simulink model "TargetPosVel"  (R2024b)
settings: Solver=ode4  StartTime=0.0  StopTime=stopTime  FixedStep=timeStep  RelTol=1e-3
values from neighbouring files (symbols this model uses):
  c = 299792458    [FMC.m]
  CD = 2.2    [FMC.m]
  dayValue = 1    [FMC.m]    (also in validation.m)
  dimx = 226.3/1000    (= 0.2263)    [FMC.m]
  dimz = 360/1000    (= 0.36)    [FMC.m]
  FL = 50e-3    (= 0.05)    [FMC.m]
  fps = 1/timeStep    (= 20)    [FMC.m]
  hourValue = 12    [FMC.m]    (also in validation.m)
  I = [Ixx Ixy Ixz; Ixy Iyy Iyz; Ixz Iyz Izz]    [FMC.m]
  I_W = [I_w 0 0; 0 I_w 0; 0 0 I_w]    [FMC.m]
  kd = 0.022    [FMC.m]
  kq = 0.0032    [FMC.m]
  L_pixel = 4.8e-6    (= 4.8e-06)    [FMC.m]
  max_h = I_w*max_speed    (= 0.00954258768528)    [FMC.m]
  max_t = 2e-3    (= 0.002)    [FMC.m]
  minuteValue = 0    [FMC.m]    (also in validation.m)
  mu_E = 3.986004418e14    (= 398600441800000)    [FMC.m]
  Omega_E = 7.2921159e-5    (= 7.2921159e-05)    [FMC.m]
  P0_Kfilter = blkdiag(eye(3), eye(3))    [FMC.m]
  Phi = 1358    [FMC.m]
  pointing_body = [0,0,1]    [FMC.m]
  q = 0.6    [FMC.m]
  Q_b = 0.05*eye(3)    [FMC.m]
  Q_LoS = 0.1*eye(3)    [FMC.m]
  quat0 = [0.6387; -0.3737; 0.6003; 0.3034]    [FMC.m]
  R_E = 6378*1000    (= 6378000)    [FMC.m]
  R_meas = norm(LoS_0)*L_pixel*fps/FL*Q_b    [FMC.m]
  rand_vec = rand_vec/norm(rand_vec)    [FMC.m]
  rcp = [0.013 0.02 0.05]    [FMC.m]
  res_dipole = 0.05    [FMC.m]
  secondValue = 0    [FMC.m]    (also in validation.m)
  sma = R_E + H    (= 6628000)    [FMC.m]
  timeStep = 0.05    [FMC.m]
  w0 = [w0x; w0y; w0z]    [FMC.m]
  x0_Kfilter = [LoS_0,;b_0]    [FMC.m]
  yearValue = 2025    [FMC.m]    (also in validation.m)
undefined symbols (not defined in the file or in its folder): IAU, WMM2020
libraries: aerolibtransform2 x14, aerolibutil x13, matrix_library x12, vrlib x5, sharedtransform x2, sharedTrackingLibrary x1, aerolibatmos2 x1, aerolibgravity2 x1, sensorgpslib x1, visionsources x1
(part 1 of 2)
settings Model: Creator=nicolasgagliardi  LastModifiedBy=nicolasgagliardi

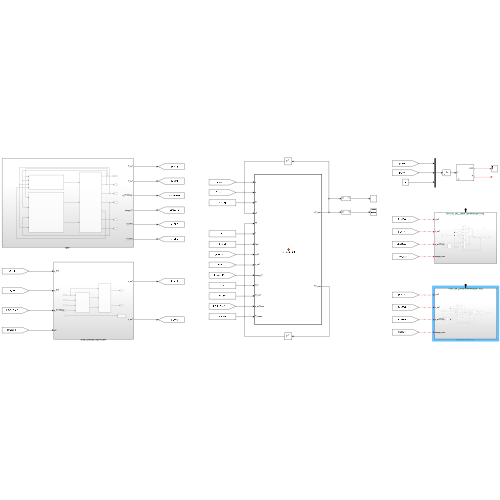
[thumbnail: Simulink's stored preview of the top-level diagram]
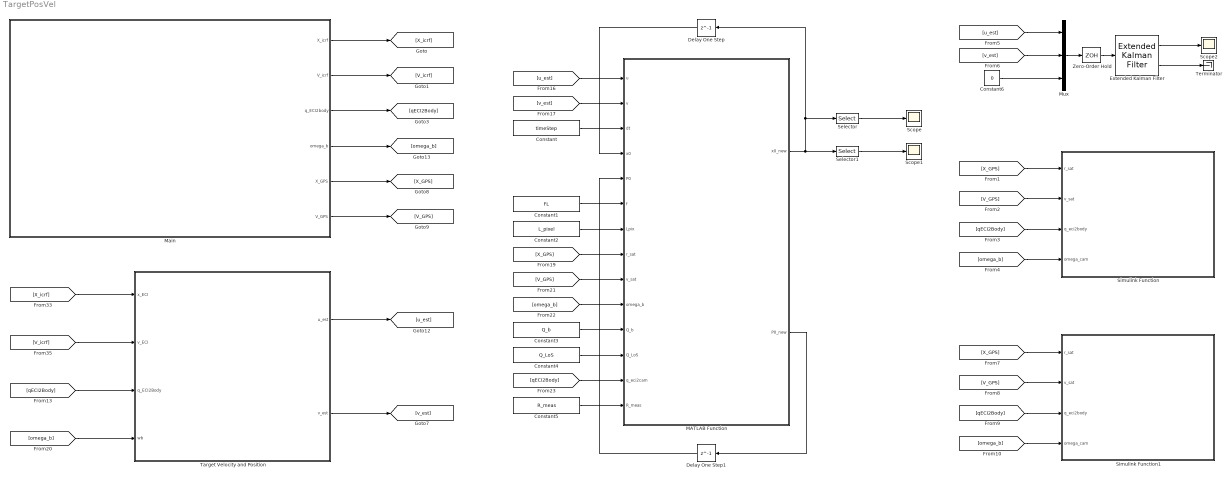
== system TargetPosVel ==
  Constant : Constant  Value=timeStep
  Constant1 : Constant  Value=FL
  Constant2 : Constant  Value=L_pixel
  Constant3 : Constant  Value=Q_b
  Constant4 : Constant  Value=Q_LoS
  Constant5 : Constant  Value=R_meas
  Constant6 : Constant  Value=0
  Delay One Step : Delay  DelayLength=1  InitialCondition=x0_Kfilter  SampleTime=timeStep
  Delay One Step1 : Delay  DelayLength=1  InitialCondition=P0_Kfilter  SampleTime=timeStep
  Extended Kalman Filter : sharedTrackingLibrary/Extended Kalman Filter  StateTransitionFcn=state_dynamics  HasStateTransitionJacobianFcn=off  HasAdditiveProcessNoise=Additive  ProcessNoise=Q_LoS  HasTimeVaryingProcessNoise=off  HasStateTransitionFcnExtraArgument=0  InitialState=x0_Kfilter(1:3)  InitialStateCovariance=P0_Kfilter(1:3,1:3)  MeasurementFcn1=measurements  HasMeasurementJacobianFcn1=off  HasMeasurementEnablePort1=off  HasAdditiveMeasurementNoise1=Additive  MeasurementNoise1=R_meas  HasTimeVaryingMeasurementNoise1=off  HasMeasurementFcnExtraArgument1=0  HasMeasurementWrapping1=off  MeasurementFcn2=myMeasurementFcn  HasMeasurementJacobianFcn2=off  HasMeasurementEnablePort2=off  HasAdditiveMeasurementNoise2=Additive  MeasurementNoise2=1  HasTimeVaryingMeasurementNoise2=off  HasMeasurementFcnExtraArgument2=0  HasMeasurementWrapping2=off  MeasurementFcn3=myMeasurementFcn  HasMeasurementJacobianFcn3=off  HasMeasurementEnablePort3=off  HasAdditiveMeasurementNoise3=Additive  MeasurementNoise3=1  HasTimeVaryingMeasurementNoise3=off  HasMeasurementFcnExtraArgument3=0  HasMeasurementWrapping3=off  MeasurementFcn4=myMeasurementFcn  HasMeasurementJacobianFcn4=off  HasMeasurementEnablePort4=off  HasAdditiveMeasurementNoise4=Additive  MeasurementNoise4=1  HasTimeVaryingMeasurementNoise4=off  HasMeasurementFcnExtraArgument4=0  HasMeasurementWrapping4=off  MeasurementFcn5=myMeasurementFcn  HasMeasurementJacobianFcn5=off  HasMeasurementEnablePort5=off  HasAdditiveMeasurementNoise5=Additive  MeasurementNoise5=1  HasTimeVaryingMeasurementNoise5=off  HasMeasurementFcnExtraArgument5=0  HasMeasurementWrapping5=off  EnableMultirate=off  StateTransitionFcnSampleTime=1  MeasurementFcn1SampleTime=1  MeasurementFcn2SampleTime=1  MeasurementFcn3SampleTime=1  MeasurementFcn4SampleTime=1  MeasurementFcn5SampleTime=1  UseCurrentEstimator=on  OutputStateCovariance=on  DataType=double  SampleTime=timeStep  NumberOfMeasurements=1
  MATLAB Function : MATLAB Function  TreatAsAtomicUnit=on
  Main : Subsystem
  Mux : Mux  Inputs=3
  Scope : Scope
  Scope1 : Scope
  Scope2 : Scope
  Selector : Selector  InputPortWidth=6  IndexOptions=Index vector (dialog)  Indices=[1 2 3]  OutputSizes=1
  Selector1 : Selector  InputPortWidth=6  IndexOptions=Index vector (dialog)  Indices=[4 5 6]  OutputSizes=1
  Simulink Function : Subsystem  TreatAsAtomicUnit=on
  Simulink Function1 : Subsystem  TreatAsAtomicUnit=on
  Target Velocity and Position : Subsystem
  Terminator : Terminator
  Zero-Order Hold : ZeroOrderHold  SampleTime=timeStep
  wires:
  [qECI2Body] -> Target Velocity and Position/3(q_ECI2Body)
  [omega_b] -> Target Velocity and Position/4(wb)
  [V_icrf] -> Target Velocity and Position/2(v_ECI)
  [X_icrf] -> Target Velocity and Position/1(x_ECI)
  Main/1(X_icrf) -> [X_icrf]
  Main/3(q_ECI2body) -> [qECI2Body]
  Main/4(omega_b) -> [omega_b]
  Main/2(V_icrf) -> [V_icrf]
  Target Velocity and Position/2(v_est) -> [v_est]
  Target Velocity and Position/1(u_est) -> [u_est]
  [u_est] -> MATLAB Function/1(u)
  [v_est] -> MATLAB Function/2(v)
  Constant/1 -> MATLAB Function/3(dt)
  [X_GPS] -> MATLAB Function/8(r_sat)
  [V_GPS] -> MATLAB Function/9(v_sat)
  [omega_b] -> MATLAB Function/10(omega_b)
  [qECI2Body] -> MATLAB Function/13(q_eci2cam)
  Constant2/1 -> MATLAB Function/7(Lpix)
  Constant1/1 -> MATLAB Function/6(f)
  MATLAB Function/1(x0_new) -> Delay One Step/1, Selector/1, Selector1/1
  MATLAB Function/2(P0_new) -> Delay One Step1/1
  Delay One Step/1 -> MATLAB Function/4(x0)
  Delay One Step1/1 -> MATLAB Function/5(P0)
  Main/5(X_GPS) -> [X_GPS]
  Main/6(V_GPS) -> [V_GPS]
  Constant3/1 -> MATLAB Function/11(Q_b)
  Constant4/1 -> MATLAB Function/12(Q_LoS)
  Constant5/1 -> MATLAB Function/14(R_meas)
  Selector/1 -> Scope/1
  Selector1/1 -> Scope1/1
  [X_GPS] -> Simulink Function/1(r_sat)
  [V_GPS] -> Simulink Function/2(v_sat)
  [qECI2Body] -> Simulink Function/3(q_eci2body)
  [omega_b] -> Simulink Function/4(omega_cam)
  Mux/1 -> Zero-Order Hold/1
  [X_GPS] -> Simulink Function1/1(r_sat)
  [V_GPS] -> Simulink Function1/2(v_sat)
  [qECI2Body] -> Simulink Function1/3(q_eci2body)
  [omega_b] -> Simulink Function1/4(omega_cam)
  Extended Kalman Filter/2 -> Terminator/1
  Extended Kalman Filter/1 -> Scope2/1
  Constant6/1 -> Mux/3
  [v_est] -> Mux/2
  [u_est] -> Mux/1
  Zero-Order Hold/1 -> Extended Kalman Filter/1

== system TargetPosVel/Main ==
  Control Torques : Subsystem
  Environmental Torques : Subsystem
  Subsystem : Subsystem
  X_icrf : Outport
  V_icrf : Outport  Port=2
  q_ECI2body : Outport  Port=3
  omega_b : Outport  Port=4
  X_GPS : Outport  Port=5
  V_GPS : Outport  Port=6
  wires:
  Subsystem/1(X_icrf) -> Environmental Torques/1(X_icrf), Control Torques/1(r_ECI), X_icrf/1
  Subsystem/2(V_icrf) -> Environmental Torques/2(V_icrf), Control Torques/2(v_ECI), V_icrf/1
  Subsystem/3(q_ECI2body) -> q_ECI2body/1, Environmental Torques/3(qECI2body), Control Torques/4(q_ECI2body)
  Subsystem/4(omega_b) -> omega_b/1, Control Torques/3(omega_b)
  Subsystem/5(t_JD) -> Environmental Torques/4(t_JD)
  Subsystem/6(X_GPS) -> X_GPS/1
  Subsystem/7(V_GPS) -> V_GPS/1
  Control Torques/1(h) -> Subsystem/2(h_rw)
  Control Torques/2(dh_dt) -> Subsystem/3(hdot_rw)
  Environmental Torques/1(T_tot) -> Subsystem/1(T_dist)

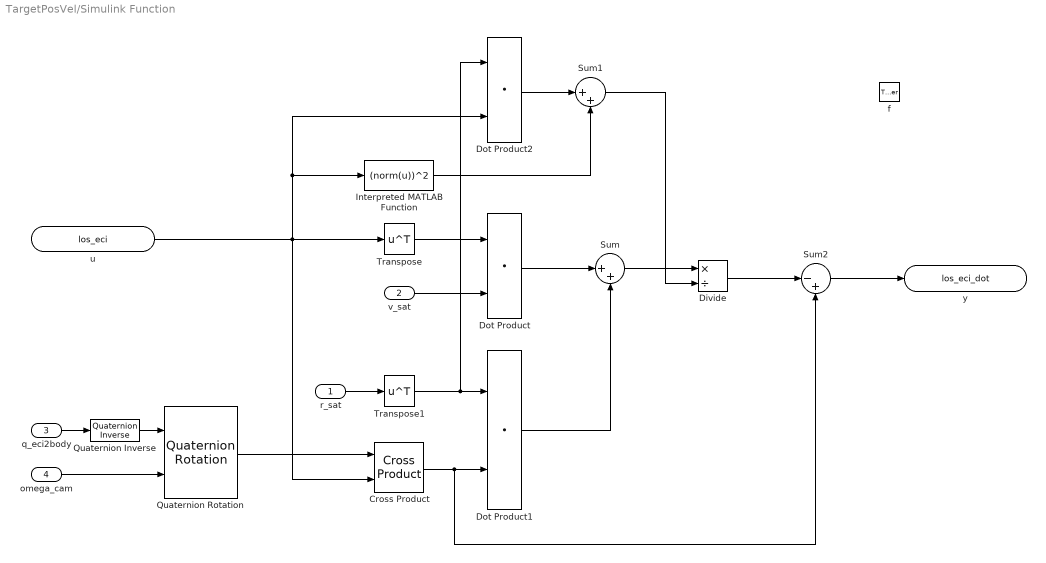
== system TargetPosVel/Simulink Function ==
  r_sat : Inport
  v_sat : Inport  Port=2
  q_eci2body : Inport  Port=3
  omega_cam : Inport  Port=4
  f : TriggerPort  TriggerType=function-call  IsSimulinkFunction=on  FunctionName=state_dynamics  FunctionVisibility=scoped  VariantControl=(inherit)
  Cross Product : matrix_library/Cross Product
  Divide : Product  Inputs=*/
  Dot Product : DotProduct  OutDataTypeStr=Inherit: Inherit via internal rule
  Dot Product1 : DotProduct  OutDataTypeStr=Inherit: Inherit via internal rule
  Dot Product2 : DotProduct  OutDataTypeStr=Inherit: Inherit via internal rule
  Interpreted MATLAB Function : MATLABFcn  MATLABFcn=(norm(u))^2
  Quaternion Inverse : aerolibutil/Quaternion Inverse
  Quaternion Rotation : aerolibutil/Quaternion Rotation
  Sum : Sum  Inputs=|++
  Sum1 : Sum  Inputs=|++
  Sum2 : Sum  Inputs=|-+
  Transpose : Math  Operator=transpose
  Transpose1 : Math  Operator=transpose
  u : ArgIn  DisableCoverage=on  PortDimensions=[3,1]  ArgumentName=los_eci
  y : ArgOut  DisableCoverage=on  PortDimensions=[3,1]  ArgumentName=los_eci_dot
  wires:
  q_eci2body/1 -> Quaternion Inverse/1
  omega_cam/1 -> Quaternion Rotation/2
  u/1 -> Transpose/1, Interpreted MATLAB Function/1, Dot Product2/2, Cross Product/2
  Transpose/1 -> Dot Product/1
  v_sat/1 -> Dot Product/2
  Dot Product/1 -> Sum/1
  r_sat/1 -> Transpose1/1
  Transpose1/1 -> Dot Product2/1, Dot Product1/1
  Quaternion Rotation/1 -> Cross Product/1
  Dot Product1/1 -> Sum/2
  Sum/1 -> Divide/1
  Dot Product2/1 -> Sum1/1
  Interpreted MATLAB Function/1 -> Sum1/2
  Sum1/1 -> Divide/2
  Divide/1 -> Sum2/1
  Cross Product/1 -> Dot Product1/2, Sum2/2
  Sum2/1 -> y/1
  Quaternion Inverse/1 -> Quaternion Rotation/1

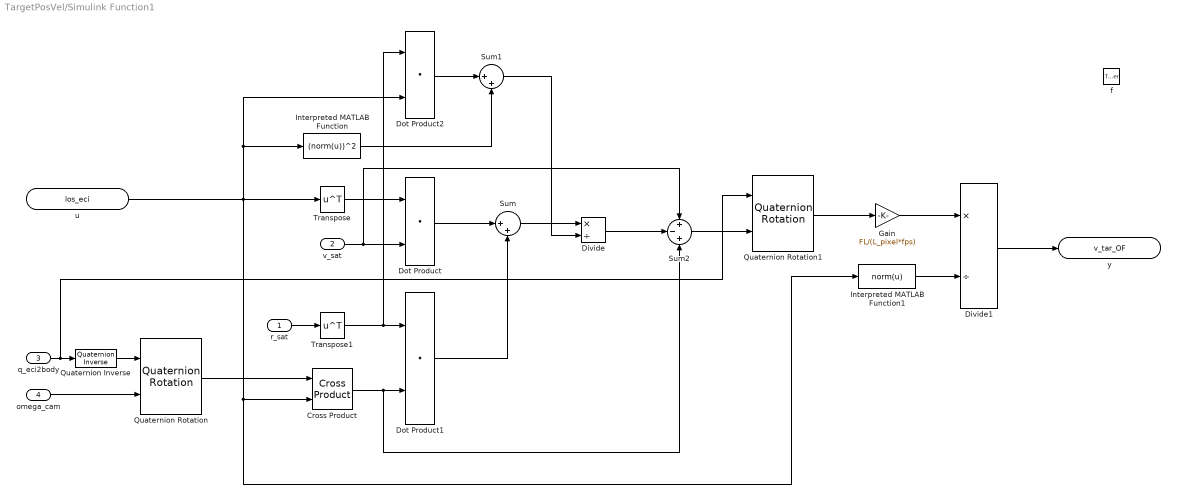
== system TargetPosVel/Simulink Function1 ==
  r_sat : Inport
  v_sat : Inport  Port=2
  q_eci2body : Inport  Port=3
  omega_cam : Inport  Port=4
  f : TriggerPort  TriggerType=function-call  IsSimulinkFunction=on  FunctionName=measurements  FunctionVisibility=scoped  VariantControl=(inherit)
  Cross Product : matrix_library/Cross Product
  Divide : Product  Inputs=*/
  Divide1 : Product  Inputs=*/
  Dot Product : DotProduct  OutDataTypeStr=Inherit: Inherit via internal rule
  Dot Product1 : DotProduct  OutDataTypeStr=Inherit: Inherit via internal rule
  Dot Product2 : DotProduct  OutDataTypeStr=Inherit: Inherit via internal rule
  Gain : Gain  Gain=FL/(L_pixel*fps)
  Interpreted MATLAB Function : MATLABFcn  MATLABFcn=(norm(u))^2
  Interpreted MATLAB Function1 : MATLABFcn  MATLABFcn=norm(u)
  Quaternion Inverse : aerolibutil/Quaternion Inverse
  Quaternion Rotation : aerolibutil/Quaternion Rotation
  Quaternion Rotation1 : aerolibutil/Quaternion Rotation
  Sum : Sum  Inputs=|++
  Sum1 : Sum  Inputs=|++
  Sum2 : Sum  Inputs=+-+
  Transpose : Math  Operator=transpose
  Transpose1 : Math  Operator=transpose
  u : ArgIn  DisableCoverage=on  PortDimensions=[3,1]  ArgumentName=los_eci
  y : ArgOut  DisableCoverage=on  PortDimensions=[3,1]  ArgumentName=v_tar_OF
  wires:
  Cross Product/1 -> Dot Product1/2, Sum2/3
  Sum1/1 -> Divide/2
  Interpreted MATLAB Function/1 -> Sum1/2
  Dot Product2/1 -> Sum1/1
  Sum/1 -> Divide/1
  Dot Product1/1 -> Sum/2
  Quaternion Rotation/1 -> Cross Product/1
  Transpose1/1 -> Dot Product1/1, Dot Product2/1
  r_sat/1 -> Transpose1/1
  Dot Product/1 -> Sum/1
  v_sat/1 -> Dot Product/2, Sum2/1
  Transpose/1 -> Dot Product/1
  u/1 -> Transpose/1, Cross Product/2, Interpreted MATLAB Function1/1, Dot Product2/2, Interpreted MATLAB Function/1
  omega_cam/1 -> Quaternion Rotation/2
  q_eci2body/1 -> Quaternion Rotation1/1, Quaternion Inverse/1
  Divide/1 -> Sum2/2
  Quaternion Inverse/1 -> Quaternion Rotation/1
  Sum2/1 -> Quaternion Rotation1/2
  Quaternion Rotation1/1 -> Gain/1
  Gain/1 -> Divide1/1
  Interpreted MATLAB Function1/1 -> Divide1/2
  Divide1/1 -> y/1

== system TargetPosVel/Target Velocity and Position ==
  x_ECI : Inport
  v_ECI : Inport  Port=2
  q_ECI2Body : Inport  Port=3
  wb : Inport  Port=4
  Clock1 : Clock
      settings: Decimation=1/timeStep
  Subsystem1 : Subsystem
  Subsystem8 : Subsystem
  To Workspace3 : ToWorkspace  VariableName=time  SampleTime=-1
      settings: Save2DSignal=2-D array (concatenate along first dimension)
  u_est : Outport
  v_est : Outport  Port=2
  wires:
  Clock1/1 -> To Workspace3/1
  q_ECI2Body/1 -> Subsystem8/1(q_ECI2body), Subsystem1/1(q_ECI2Body)
  v_ECI/1 -> Subsystem8/2(v_S/C)
  x_ECI/1 -> Subsystem8/3(r_S/C)
  wb/1 -> Subsystem8/4(wb)
  Subsystem8/2(vP_ECEF) -> Subsystem1/3(vP_ECEF)
  Subsystem8/1(rho) -> Subsystem1/2(rho)
  Subsystem1/1(u_est) -> u_est/1
  Subsystem1/2(v_est) -> v_est/1

== system TargetPosVel/Main/Control Torques ==
  r_ECI : Inport
  v_ECI : Inport  Port=2
  omega_b : Inport  Port=3
  q_ECI2body : Inport  Port=4
  Nadir Pointing : Subsystem  TreatAsAtomicUnit=on
  Nadir pointing : Subsystem
  RW Saturation : Subsystem
  h : Outport
  dh_dt : Outport  Port=2
  wires:
  omega_b/1 -> Nadir pointing/2(omega_b), RW Saturation/2(omega)
  RW Saturation/2(dh_dt) -> dh_dt/1
  RW Saturation/1(h) -> h/1
  Nadir pointing/1(g) -> RW Saturation/1(g)
  Nadir Pointing/1(q_Err) -> Nadir pointing/1(qErr)
  Nadir Pointing/2(w_des) -> Nadir pointing/3(omega_des_b)
  r_ECI/1 -> Nadir Pointing/1(r_ECI)
  v_ECI/1 -> Nadir Pointing/2(v_ECI)
  q_ECI2body/1 -> Nadir Pointing/3(q_ECI2body)

== system TargetPosVel/Main/Environmental Torques ==
  X_icrf : Inport
  V_icrf : Inport  Port=2
  qECI2body : Inport  Port=3
  t_JD : Inport  Port=4
  Add : Sum  Inputs=++++
  "Aerodynamic Torque  " : Subsystem
  Gravity Gradient Torque : Subsystem
  Magnetic Torque : Subsystem
  Quaternions to Direction Cosine Matrix : sharedtransform/Quaternions to  Direction Cosine Matrix  aMode=aMode
  Solar Radiation Pressure Torque : Subsystem
  T_tot : Outport
  wires:
  "Aerodynamic Torque  "/1(Tdrag) -> Add/2
  Quaternions to Direction Cosine Matrix/1 -> Magnetic Torque/2(DCM_eci2body), Solar Radiation Pressure Torque/1(DCM_eci2body), "Aerodynamic Torque  "/2(DCM_eci2body), Gravity Gradient Torque/1(DCM_eci2body)
  Gravity Gradient Torque/1(Tgg) -> Add/1
  X_icrf/1 -> Solar Radiation Pressure Torque/2(X_icrf), Magnetic Torque/1(X_icrf), "Aerodynamic Torque  "/1(X_icrf), Gravity Gradient Torque/2(X_icrf)
  V_icrf/1 -> "Aerodynamic Torque  "/3(V_icrf)
  Solar Radiation Pressure Torque/1(T_srp) -> Add/3
  qECI2body/1 -> Quaternions to Direction Cosine Matrix/1
  t_JD/1 -> Solar Radiation Pressure Torque/3(t_JD)
  Magnetic Torque/1(Tmag) -> Add/4
  Add/1 -> T_tot/1

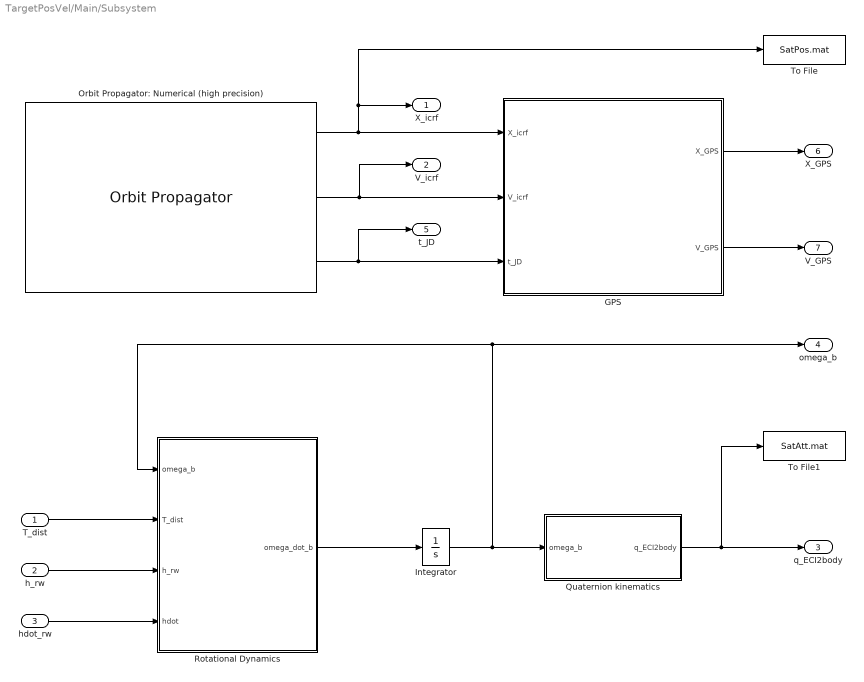
== system TargetPosVel/Main/Subsystem ==
  T_dist : Inport
  h_rw : Inport  Port=2
  hdot_rw : Inport  Port=3
  GPS : Subsystem
  Integrator : Integrator  InitialCondition=w0
  Orbit Propagator: Numerical (high precision) : OrbitPropagator  propagator=Numerical (high precision)  startDate=jdate  mass=mass  action=None  semiMajorAxis=sma  eccentricity=ecc  inclination=inc_SSO  raan=RAAN  argPeriapsis=aop  trueAnomaly=truean  inertialPosition=[3649700.0 3308200.0 -4676600.0]  inertialVelocity=[-2750.8 6666.4 2573.4]  fixedPosition=[-4142689.0 -2676864.7 -4669861.6]  fixedVelocity=[1452.7 -6720.7 2568.1]  customR=3396200  customMu=4.305e13  customJ2=1.0826269e-03  customOmega=4.06125949e-3  F107ExtrapMethod=Least squares fit  MagneticIndexExtrapMethod=IGRF  dragCoeff=CD  dragArea=dimx*dimz  useEphemerisDateRange=off  ephemerisStartDate=jdate  ephemerisEndDate=jdate  includeSunGravity=off  reflectivityCoeff=q  srpArea=dimx*dimz
  Quaternion kinematics : Subsystem
  Rotational Dynamics : Subsystem
  To File : ToFile  Filename=SatPos.mat  MatrixName=SatPos  SampleTime=timeStep
  To File1 : ToFile  Filename=SatAtt.mat  MatrixName=SatAtt  SampleTime=timeStep
  X_icrf : Outport
  V_icrf : Outport  Port=2
  q_ECI2body : Outport  Port=3
  omega_b : Outport  Port=4
  t_JD : Outport  Port=5
  X_GPS : Outport  Port=6
  V_GPS : Outport  Port=7
  wires:
  Orbit Propagator: Numerical (high precision)/3 -> t_JD/1, GPS/3(t_JD)
  Integrator/1 -> Quaternion kinematics/1(omega_b), omega_b/1, Rotational Dynamics/1(omega_b)
  GPS/1(X_GPS) -> X_GPS/1
  GPS/2(V_GPS) -> V_GPS/1
  Orbit Propagator: Numerical (high precision)/1 -> GPS/1(X_icrf), X_icrf/1, To File/1
  T_dist/1 -> Rotational Dynamics/2(T_dist)
  Rotational Dynamics/1(omega_dot_b) -> Integrator/1
  h_rw/1 -> Rotational Dynamics/3(h_rw)
  Orbit Propagator: Numerical (high precision)/2 -> V_icrf/1, GPS/2(V_icrf)
  hdot_rw/1 -> Rotational Dynamics/4(hdot)
  Quaternion kinematics/1(q_ECI2body) -> q_ECI2body/1, To File1/1

== system TargetPosVel/Target Velocity and Position/Subsystem1 ==
  q_ECI2Body : Inport
  rho : Inport  Port=2
  vP_ECEF : Inport  Port=3
  Selector2 : Selector  InputPortWidth=3  IndexOptions=Index vector (dialog)  Indices=[1 2]  OutputSizes=1
  Subsystem : Subsystem
  Subsystem4 : Subsystem
  u_est : Outport
  v_est : Outport  Port=2
  wires:
  q_ECI2Body/1 -> Subsystem/2(q_ECI2Body)
  vP_ECEF/1 -> Subsystem/1(vP_ECEF)
  rho/1 -> Subsystem4/2(rho)
  Subsystem4/2(v_est) -> v_est/1
  Subsystem4/1(u_est) -> u_est/1
  Subsystem/1(vP_body) -> Selector2/1
  Selector2/1 -> Subsystem4/1(vP)

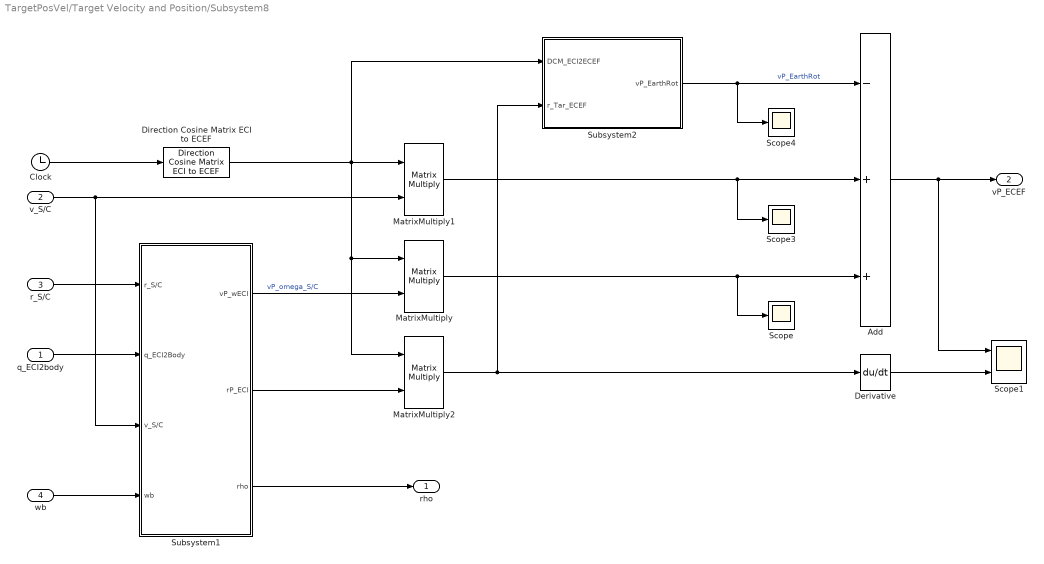
== system TargetPosVel/Target Velocity and Position/Subsystem8 ==
  q_ECI2body : Inport
  v_S/C : Inport  Port=2
  r_S/C : Inport  Port=3
  wb : Inport  Port=4
  Add : Sum  Inputs=-++
  Clock : Clock
  Derivative : Derivative
  Direction Cosine Matrix ECI to ECEF : aerolibtransform2/Direction Cosine Matrix ECI to ECEF  red=IAU-2000/2006  year=yearValue  month=January  day=1  hour=hourValue  min=minuteValue  sec=secondValue  deltaT=Sec  errorflag=Error  extraparamflag=off
      settings: AttributesFormatString=%<red>
  MatrixMultiply : Product  Multiplication=Matrix(*)
  MatrixMultiply1 : Product  Multiplication=Matrix(*)
  MatrixMultiply2 : Product  Multiplication=Matrix(*)
  Scope : Scope
  Scope1 : Scope  NumInputPorts=2
  Scope3 : Scope
  Scope4 : Scope
  Subsystem1 : Subsystem
  Subsystem2 : Subsystem
  rho : Outport
  vP_ECEF : Outport  Port=2
  wires:
  r_S/C/1 -> Subsystem1/1(r_S/C)
  Subsystem2/1(vP_EarthRot) -> Add/1, Scope4/1  "vP_EarthRot"
  Add/1 -> vP_ECEF/1, Scope1/1
  Subsystem1/1(vP_wECI) -> MatrixMultiply/2  "vP_omega_S/C"
  Subsystem1/2(rP_ECI) -> MatrixMultiply2/2
  q_ECI2body/1 -> Subsystem1/2(q_ECI2Body)
  wb/1 -> Subsystem1/4(wb)
  v_S/C/1 -> MatrixMultiply1/2, Subsystem1/3(v_S/C)
  Clock/1 -> Direction Cosine Matrix ECI to ECEF/1
  MatrixMultiply/1 -> Scope/1, Add/3
  MatrixMultiply1/1 -> Add/2, Scope3/1
  MatrixMultiply2/1 -> Subsystem2/2(r_Tar_ECEF), Derivative/1
  Direction Cosine Matrix ECI to ECEF/1 -> Subsystem2/1(DCM_ECI2ECEF), MatrixMultiply1/1, MatrixMultiply2/1, MatrixMultiply/1
  Subsystem1/3(rho) -> rho/1
  Derivative/1 -> Scope1/2

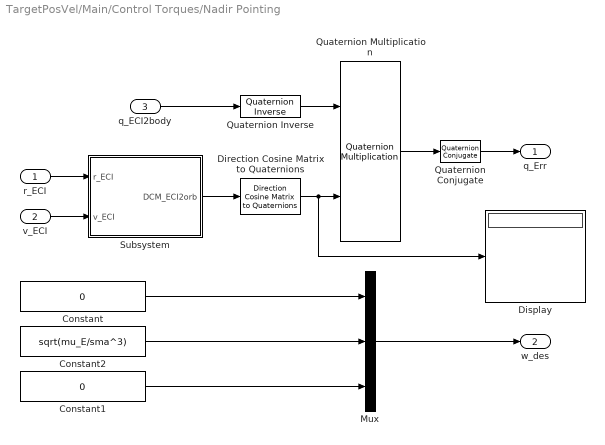
== system TargetPosVel/Main/Control Torques/Nadir Pointing ==
  r_ECI : Inport
  v_ECI : Inport  Port=2
  q_ECI2body : Inport  Port=3
  Constant : Constant  Value=0
  Constant1 : Constant  Value=0
  Constant2 : Constant  Value=sqrt(mu_E/sma^3)
  Direction Cosine Matrix to Quaternions : sharedtransform/Direction Cosine Matrix  to Quaternions  aMode=0  action=None  tolerance=eps(2)
  Display : Display
  Mux : Mux  Inputs=3
  Quaternion Conjugate : aerolibutil/Quaternion Conjugate
  Quaternion Inverse : aerolibutil/Quaternion Inverse
  Quaternion Multiplication : aerolibutil/Quaternion Multiplication
  Subsystem : Subsystem
  q_Err : Outport
  w_des : Outport  Port=2
  wires:
  Quaternion Multiplication/1 -> Quaternion Conjugate/1
  q_ECI2body/1 -> Quaternion Inverse/1
  Constant2/1 -> Mux/2
  Constant1/1 -> Mux/3
  Constant/1 -> Mux/1
  Mux/1 -> w_des/1
  Quaternion Inverse/1 -> Quaternion Multiplication/1
  Direction Cosine Matrix to Quaternions/1 -> Display/1, Quaternion Multiplication/2
  Quaternion Conjugate/1 -> q_Err/1
  v_ECI/1 -> Subsystem/2(v_ECI)
  Subsystem/1(DCM_ECI2orb) -> Direction Cosine Matrix to Quaternions/1
  r_ECI/1 -> Subsystem/1(r_ECI)

== system TargetPosVel/Main/Control Torques/Nadir pointing ==
  qErr : Inport
  omega_b : Inport  Port=2
  omega_des_b : Inport  Port=3
  Add2 : Sum  Inputs=+-
  Gain2 : Gain  Gain=kq
  Gain3 : Gain  Gain=kd
  Product1 : Product
  Selector3 : Selector  InputPortWidth=4  IndexOptions=Index vector (dialog)  Indices=[2 3 4]  OutputSizes=1
  Selector4 : Selector  InputPortWidth=4  IndexOptions=Index vector (dialog)  Indices=[1]  OutputSizes=1
  Sum2 : Sum
  g : Outport
  wires:
  Gain3/1 -> Sum2/2
  Gain2/1 -> Product1/2
  Add2/1 -> Gain3/1
  Selector4/1 -> Product1/1
  qErr/1 -> Selector3/1, Selector4/1
  Selector3/1 -> Gain2/1
  omega_des_b/1 -> Add2/2
  Sum2/1 -> g/1
  Product1/1 -> Sum2/1
  omega_b/1 -> Add2/1

== system TargetPosVel/Main/Control Torques/RW Saturation ==
  g : Inport
  omega : Inport  Port=2
  Add : Sum  Inputs=+-
  Constant : Constant  Value=I_W
  Derivative : Derivative
  Derivative1 : Derivative
  Integrator : Integrator  InitialCondition=zeros(3,1)
  Integrator1 : Integrator  InitialCondition=zeros(3,1)
  Product : Product  Multiplication=Matrix(*)
  Saturation : Saturate  UpperLimit=[max_t;max_t;max_t]  LowerLimit=-[max_t;max_t;max_t]
  Saturation1 : Saturate  UpperLimit=[max_h;max_h;max_h]  LowerLimit=-[max_h;max_h;max_h]
  h : Outport
  dh_dt : Outport  Port=2
  wires:
  omega/1 -> Derivative/1
  Constant/1 -> Product/1
  g/1 -> Add/1
  Product/1 -> Add/2
  Derivative/1 -> Product/2
  Integrator/1 -> h/1
  Derivative1/1 -> Saturation/1
  Integrator1/1 -> Saturation1/1  "h"
  Saturation1/1 -> Derivative1/1
  Saturation/1 -> Integrator/1, dh_dt/1
  Add/1 -> Integrator1/1  "hdot"

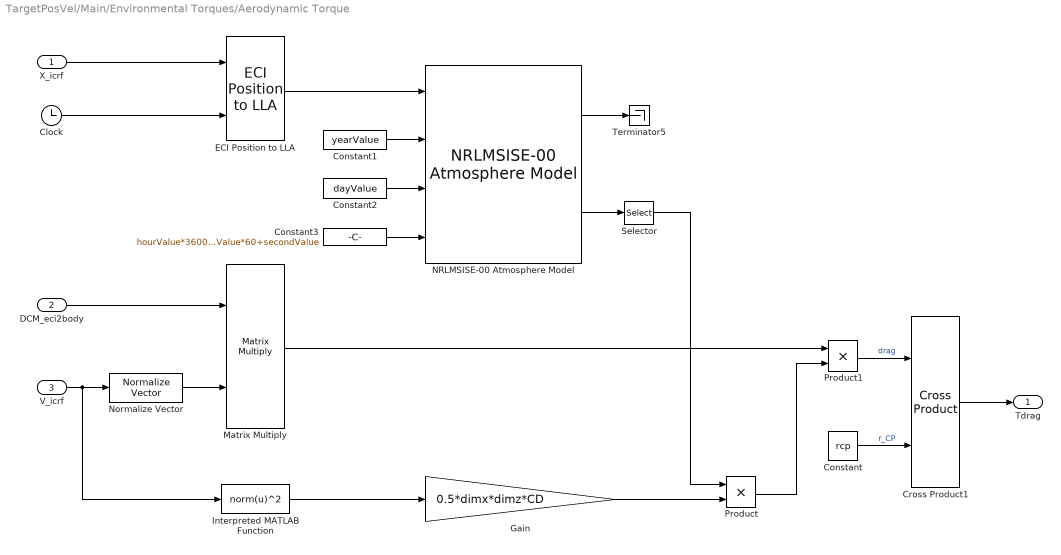
== system TargetPosVel/Main/Environmental Torques/Aerodynamic Torque   ==
  X_icrf : Inport
  DCM_eci2body : Inport  Port=2
  V_icrf : Inport  Port=3
  Clock : Clock
  Constant : Constant  Value=rcp
  Constant1 : Constant  Value=yearValue
  Constant2 : Constant  Value=dayValue
  Constant3 : Constant  Value=hourValue*3600+minuteValue*60+secondValue
  Cross Product1 : matrix_library/Cross Product
  ECI Position to LLA : aerolibtransform2/ECI Position to LLA  red=IAU-2000/2006  year=yearValue  month=January  day=1  hour=hourValue  min=minuteValue  sec=secondValue  deltaT=Sec  errorflag=Warning  extraparamflag=off  eunits=Metric (MKS)  earthmodel=WGS84  flat=1/298.257223563  eqradius=6378137
      settings: AttributesFormatString=%<red>
  Gain : Gain  Gain=0.5*dimx*dimz*CD
  Interpreted MATLAB Function : MATLABFcn  MATLABFcn=norm(u)^2
  Matrix Multiply : Product  Multiplication=Matrix(*)
  NRLMSISE-00 Atmosphere Model : aerolibatmos2/NRLMSISE-00 Atmosphere Model  units=Metric (MKS)  lst_input=off  flux_ap_input=off  flags_input=Internal  flags=ones(1,23)  oxygen_in=off  action=None
  Normalize Vector : vrlib/Utilities/Normalize Vector  maxzero=0
  Product : Product
  Product1 : Product
  Selector : Selector  InputPortWidth=9  IndexOptions=Index vector (dialog)  Indices=6  OutputSizes=1
  Terminator5 : Terminator
  Tdrag : Outport
  wires:
  X_icrf/1 -> ECI Position to LLA/1
  Gain/1 -> Product/2
  V_icrf/1 -> Interpreted MATLAB Function/1, Normalize Vector/1
  Interpreted MATLAB Function/1 -> Gain/1
  DCM_eci2body/1 -> Matrix Multiply/1
  Normalize Vector/1 -> Matrix Multiply/2
  Matrix Multiply/1 -> Product1/1
  Product/1 -> Product1/2
  Cross Product1/1 -> Tdrag/1
  Clock/1 -> ECI Position to LLA/2
  Product1/1 -> Cross Product1/1  "drag"
  Constant/1 -> Cross Product1/2  "r_CP"
  Constant1/1 -> NRLMSISE-00 Atmosphere Model/2
  Constant3/1 -> NRLMSISE-00 Atmosphere Model/4
  ECI Position to LLA/1 -> NRLMSISE-00 Atmosphere Model/1
  Constant2/1 -> NRLMSISE-00 Atmosphere Model/3
  NRLMSISE-00 Atmosphere Model/2 -> Selector/1
  NRLMSISE-00 Atmosphere Model/1 -> Terminator5/1
  Selector/1 -> Product/1

== system TargetPosVel/Main/Environmental Torques/Gravity Gradient Torque ==
  DCM_eci2body : Inport
  X_icrf : Inport  Port=2
  Constant : Constant  Value=I
  Cross Product : matrix_library/Cross Product
  Divide : Product  Inputs=*/
  Gain : Gain  Gain=3*mu_E
  Interpreted MATLAB Function : MATLABFcn  MATLABFcn=norm(u)^3
  Matrix Multiply : Product  Multiplication=Matrix(*)
  Matrix Multiply2 : Product  Multiplication=Matrix(*)
  Normalize Vector1 : vrlib/Utilities/Normalize Vector  maxzero=0
  Tgg : Outport
  wires:
  X_icrf/1 -> Interpreted MATLAB Function/1, Matrix Multiply/2
  Normalize Vector1/1 -> Matrix Multiply2/2, Cross Product/1
  Divide/1 -> Tgg/1
  Matrix Multiply/1 -> Normalize Vector1/1
  Gain/1 -> Divide/1
  Matrix Multiply2/1 -> Cross Product/2
  Constant/1 -> Matrix Multiply2/1
  DCM_eci2body/1 -> Matrix Multiply/1
  Interpreted MATLAB Function/1 -> Divide/2  "Rs^3"
  Cross Product/1 -> Gain/1

== system TargetPosVel/Main/Environmental Torques/Magnetic Torque ==
  X_icrf : Inport
  DCM_eci2body : Inport  Port=2
  Clock : Clock
  Constant : Constant  Value=res_dipole
  Constant1 : Constant  Value=rand_vec
  Cross Product2 : matrix_library/Cross Product
  Direction Cosine Matrix ECI to ECEF : aerolibtransform2/Direction Cosine Matrix ECI to ECEF  red=IAU-2000/2006  year=yearValue  month=January  day=1  hour=hourValue  min=minuteValue  sec=secondValue  deltaT=Sec  errorflag=Error  extraparamflag=off
      settings: AttributesFormatString=%<red>
  MatrixMultiply : Product  Multiplication=Matrix(*)
  Product : Product
  Product4 : Product  Multiplication=Matrix(*)
  Subsystem : Subsystem
  Transpose : Math  Operator=transpose
  Tmag : Outport
  wires:
  Product4/1 -> Tmag/1
  Constant/1 -> Product/1
  Product/1 -> Cross Product2/1
  DCM_eci2body/1 -> Product4/1
  Constant1/1 -> Product/2
  MatrixMultiply/1 -> Cross Product2/2  "MagField_ECI"
  Cross Product2/1 -> Product4/2  "Tmag_ECI"
  X_icrf/1 -> Subsystem/1(Xi)
  Subsystem/1(MagField_ECEF) -> MatrixMultiply/2
  Clock/1 -> Direction Cosine Matrix ECI to ECEF/1
  Transpose/1 -> MatrixMultiply/1
  Direction Cosine Matrix ECI to ECEF/1 -> Transpose/1

== system TargetPosVel/Main/Environmental Torques/Solar Radiation Pressure Torque ==
  DCM_eci2body : Inport
  X_icrf : Inport  Port=2
  t_JD : Inport  Port=3
  Add2 : Sum  Inputs=-+
  Constant : Constant  Value=rcp
  Cross Product3 : matrix_library/Cross Product
  Gain3 : Gain  Gain=-Phi*dimx*dimz*(1+q)/c
  Matrix Multiply4 : Product  Multiplication=Matrix(*)
  Normalize Vector2 : vrlib/Utilities/Normalize Vector  maxzero=0
  Planetary Ephemeris : PlanetaryEphem  units=m,m/s  target=Sun  outputVelocity=off
  T_srp : Outport
  wires:
  Gain3/1 -> Cross Product3/2
  Add2/1 -> Normalize Vector2/1
  Normalize Vector2/1 -> Matrix Multiply4/2
  Matrix Multiply4/1 -> Gain3/1
  X_icrf/1 -> Add2/1
  t_JD/1 -> Planetary Ephemeris/1
  Cross Product3/1 -> T_srp/1
  Constant/1 -> Cross Product3/1
  DCM_eci2body/1 -> Matrix Multiply4/1
  Planetary Ephemeris/1 -> Add2/2  "Xi_SUN"

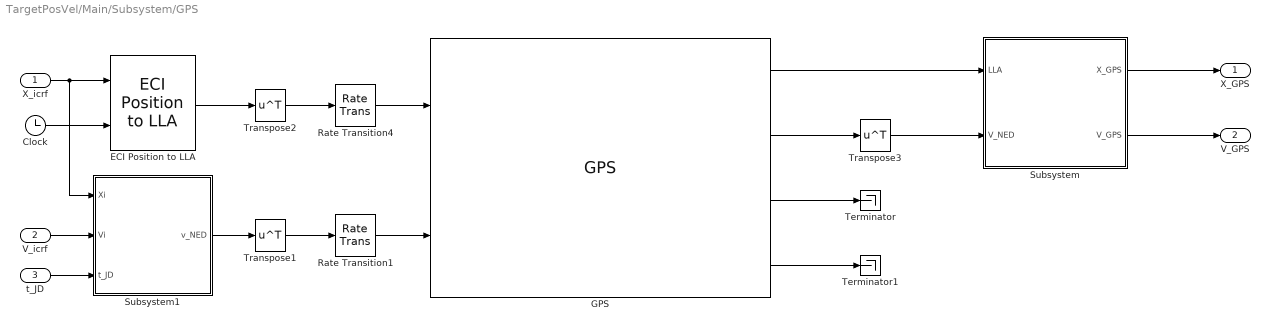
== system TargetPosVel/Main/Subsystem/GPS ==
  X_icrf : Inport
  V_icrf : Inport  Port=2
  t_JD : Inport  Port=3
  Clock : Clock
  ECI Position to LLA : aerolibtransform2/ECI Position to LLA  red=IAU-2000/2006  year=yearValue  month=January  day=1  hour=hourValue  min=minuteValue  sec=secondValue  deltaT=Sec  errorflag=Error  extraparamflag=off  eunits=Metric (MKS)  earthmodel=WGS84  flat=1/298.257223563  eqradius=6378137
      settings: AttributesFormatString=%<red>
  GPS : sensorgpslib/GPS  DispRefFrame=NED  PositionInputFormat=Geodetic  ReferenceLocation=[ 0, 0, 0 ]  HorizontalPositionAccuracy=GPSHAccuracy  VerticalPositionAccuracy=GPSVAccuracy  VelocityAccuracy=GPSVelAccuracy  DecayFactor=0  SeedDouble=67  SimulateUsing=Interpreted execution
  Rate Transition1 : RateTransition  OutPortSampleTime=timeStep*10
  Rate Transition4 : RateTransition  OutPortSampleTime=timeStep*10
  Subsystem : Subsystem
  Subsystem1 : Subsystem
  Terminator : Terminator
  Terminator1 : Terminator
  Transpose1 : Math  Operator=transpose
  Transpose2 : Math  Operator=transpose
  Transpose3 : Math  Operator=transpose
  X_GPS : Outport
  V_GPS : Outport  Port=2
  wires:
  V_icrf/1 -> Subsystem1/2(Vi)
  Subsystem1/1(v_NED) -> Transpose1/1
  ECI Position to LLA/1 -> Transpose2/1
  Rate Transition4/1 -> GPS/1
  Rate Transition1/1 -> GPS/2
  Transpose1/1 -> Rate Transition1/1
  Transpose2/1 -> Rate Transition4/1
  X_icrf/1 -> Subsystem1/1(Xi), ECI Position to LLA/1
  GPS/3 -> Terminator/1
  GPS/4 -> Terminator1/1
  t_JD/1 -> Subsystem1/3(t_JD)
  GPS/2 -> Transpose3/1
  GPS/1 -> Subsystem/1(LLA)
  Transpose3/1 -> Subsystem/2(V_NED)
  Subsystem/2(V_GPS) -> V_GPS/1
  Clock/1 -> ECI Position to LLA/2
  Subsystem/1(X_GPS) -> X_GPS/1

== system TargetPosVel/Main/Subsystem/Quaternion kinematics ==
  omega_b : Inport
  Gain1 : Gain  Gain=0.5
  Integrator1 : Integrator  InitialCondition=quat0
  MATLAB Function : MATLAB Function  TreatAsAtomicUnit=on
  Product : Product  Multiplication=Matrix(*)
  q_ECI2body : Outport
  wires:
  Gain1/1 -> Product/1
  omega_b/1 -> MATLAB Function/1(omega)
  MATLAB Function/1(OMEGA) -> Gain1/1
  Integrator1/1 -> q_ECI2body/1, Product/2
  Product/1 -> Integrator1/1

== system TargetPosVel/Main/Subsystem/Rotational Dynamics ==
  omega_b : Inport
  T_dist : Inport  Port=2
  h_rw : Inport  Port=3
  hdot : Inport  Port=4
  Constant : Constant  Value=I
  Cross Product : matrix_library/Cross Product
  Invert 3x3 Matrix : aerolibutil/Invert  3x3 Matrix
  MatrixMultiply : Product  Multiplication=Matrix(*)
  MatrixMultiply1 : Product  Multiplication=Matrix(*)
  Minus : Sum  Inputs=+--
  Minus1 : Sum
  omega_dot_b : Outport
  wires:
  Invert 3x3 Matrix/1 -> MatrixMultiply1/1
  T_dist/1 -> Minus/1
  Minus1/1 -> Cross Product/2
  MatrixMultiply1/1 -> omega_dot_b/1
  Minus/1 -> MatrixMultiply1/2
  Constant/1 -> Invert 3x3 Matrix/1, MatrixMultiply/1
  omega_b/1 -> Cross Product/1, MatrixMultiply/2
  MatrixMultiply/1 -> Minus1/1
  Cross Product/1 -> Minus/2
  h_rw/1 -> Minus1/2
  hdot/1 -> Minus/3

== system TargetPosVel/Target Velocity and Position/Subsystem1/Subsystem ==
  vP_ECEF : Inport
  q_ECI2Body : Inport  Port=2
  Clock : Clock
  Direction Cosine Matrix ECI to ECEF : aerolibtransform2/Direction Cosine Matrix ECI to ECEF  red=IAU-2000/2006  year=yearValue  month=January  day=1  hour=hourValue  min=minuteValue  sec=secondValue  deltaT=Sec  errorflag=Error  extraparamflag=off
      settings: AttributesFormatString=%<red>
  MatrixMultiply : Product  Multiplication=Matrix(*)
  Quaternion Rotation : aerolibutil/Quaternion Rotation
  Transpose : Math  Operator=transpose
  vP_body : Outport
  wires:
  Direction Cosine Matrix ECI to ECEF/1 -> Transpose/1
  Clock/1 -> Direction Cosine Matrix ECI to ECEF/1
  Transpose/1 -> MatrixMultiply/1
  vP_ECEF/1 -> MatrixMultiply/2
  MatrixMultiply/1 -> Quaternion Rotation/2
  q_ECI2Body/1 -> Quaternion Rotation/1
  Quaternion Rotation/1 -> vP_body/1

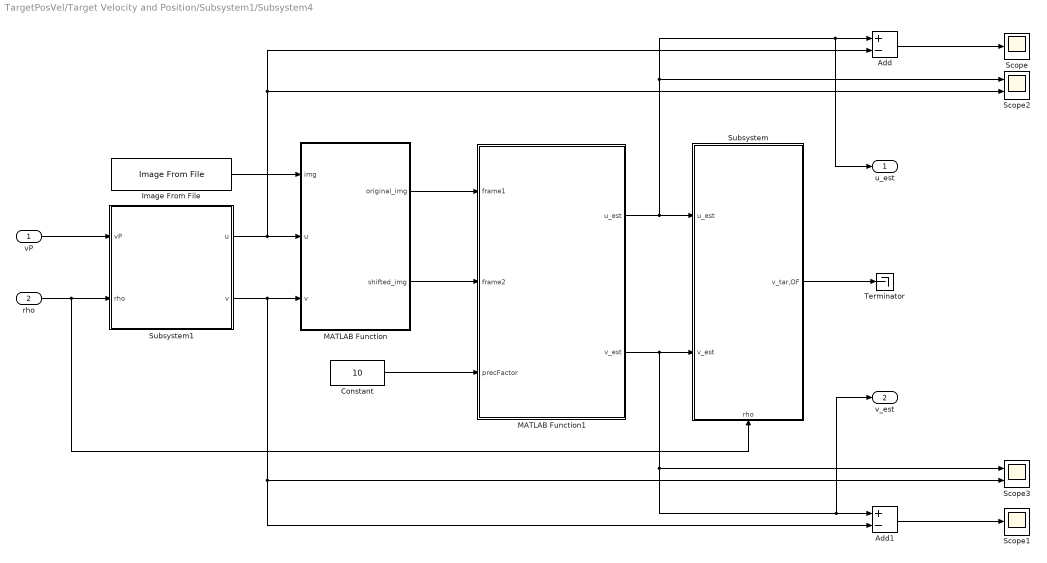
== system TargetPosVel/Target Velocity and Position/Subsystem1/Subsystem4 ==
  vP : Inport
  rho : Inport  Port=2
  Add : Sum  Inputs=+-
  Add1 : Sum  Inputs=+-
  Constant : Constant  Value=10
  Image From File : visionsources/Image From File  Tag=vipblks_nd  FileName=frame.jpg  Ts=inf  imagePorts=One multidimensional signal  OutPortLabels=R|G|B  ImageDataType=Inherit from input image  sdImageDataType=uint(8)  Signed=on  WordLength=16  FractionLengthMode=User-defined  FractionLength=15
  MATLAB Function : MATLAB Function  TreatAsAtomicUnit=on
  MATLAB Function1 : MATLAB Function  TreatAsAtomicUnit=on
  Scope : Scope
  Scope1 : Scope
  Scope2 : Scope  NumInputPorts=2
  Scope3 : Scope  NumInputPorts=2
  Subsystem : Subsystem
      settings: PortSchema="{\"entries\":[{\"content\":{\"sides\":[{\"content\":{\"connectorIds\":[\"In1\",\"In2\"]},\"type\":\"ConnectorPlacement.EquallySpacedRectSide\",\"uuid\":\"2f83bb02-0479-4d57-905b-937e4b717ae3\"},{\"content\":{\"connectorIds\":[\"Out1\"],\"side\":\"RIGHT\"},\"type\":\"ConnectorPlacement.EquallySpacedRectSide\",\"uuid\":\"e91fda81-fd69-49ed-9639-ccd658328381\"},{\"content\":{\"side\":\"TOP\"},\"type\":\"ConnectorPlacement.EquallySpacedRectSide\",\"uuid\":\"9babdf23-9593-460b-b3fb-e1b72397bd2a\"},{\"content\":{\"connectorIds\":[\"In3\"],\"side\":\"BOTTOM\"},\"type\":\"ConnectorPlacement.EquallySpacedRectSide\",\"uuid\":\"45498332-a18a-4522-be58-a96a6bf7f645\"}]},\"type\":\"ConnectorPlacement.EquallySpacedConnector\",\"uuid\":\"6be0988f-0aad-40ec-a9ec-1a784c9f3227\"}],\"packageUris\":[\"http://schema.mathworks.com/mf0/Connector/R2020b\"],\"version\":\"1.0\"}"
  Subsystem1 : Subsystem
  Terminator : Terminator
  u_est : Outport
  v_est : Outport  Port=2
  wires:
  MATLAB Function/1(original_img) -> MATLAB Function1/1(frame1)
  MATLAB Function/2(shifted_img) -> MATLAB Function1/2(frame2)
  Image From File/1 -> MATLAB Function/1(img)
  MATLAB Function1/1(u_est) -> Scope2/1, Add/1, u_est/1, Subsystem/1(u_est)
  MATLAB Function1/2(v_est) -> Scope3/1, Add1/1, v_est/1, Subsystem/2(v_est)
  Constant/1 -> MATLAB Function1/3(precFactor)
  Subsystem/1(v_tar,OF) -> Terminator/1
  vP/1 -> Subsystem1/1(vP)
  rho/1 -> Subsystem1/2(rho), Subsystem/3(rho)
  Subsystem1/1(u) -> Scope2/2, Add/2, MATLAB Function/2(u)
  Subsystem1/2(v) -> Scope3/2, Add1/2, MATLAB Function/3(v)
  Add/1 -> Scope/1
  Add1/1 -> Scope1/1

== system TargetPosVel/Target Velocity and Position/Subsystem8/Subsystem1 ==
  r_S/C : Inport
  q_ECI2Body : Inport  Port=2
  v_S/C : Inport  Port=3
  wb : Inport  Port=4
  Subsystem : Subsystem
  Subsystem3 : Subsystem
  vP_wECI : Outport
  rP_ECI : Outport  Port=2
  rho : Outport  Port=3
  wires:
  r_S/C/1 -> Subsystem3/1(r_S/C)
  v_S/C/1 -> Subsystem3/3(v_S/C)
  wb/1 -> Subsystem3/4(wb)
  Subsystem3/2(rP_ECI) -> Subsystem/1(Xi)
  q_ECI2Body/1 -> Subsystem3/2(q_ECI2Body)
  Subsystem/1(rP_ECI) -> rP_ECI/1
  Subsystem3/1(vP_wECI) -> vP_wECI/1
  Subsystem3/3(rho) -> rho/1

== system TargetPosVel/Target Velocity and Position/Subsystem8/Subsystem2 ==
  DCM_ECI2ECEF : Inport
  r_Tar_ECEF : Inport  Port=2
  Constant : Constant  Value=0
  Constant1 : Constant  Value=Omega_E
  Constant2 : Constant  Value=0
  Cross Product : matrix_library/Cross Product
  MatrixMultiply : Product  Multiplication=Matrix(*)
  Mux : Mux  Inputs=3
  vP_EarthRot : Outport
  wires:
  Constant2/1 -> Mux/2
  Constant/1 -> Mux/1
  Constant1/1 -> Mux/3
  Cross Product/1 -> vP_EarthRot/1
  r_Tar_ECEF/1 -> Cross Product/2
  Mux/1 -> MatrixMultiply/2
  MatrixMultiply/1 -> Cross Product/1
  DCM_ECI2ECEF/1 -> MatrixMultiply/1

== system TargetPosVel/Main/Control Torques/Nadir Pointing/Subsystem ==
  r_ECI : Inport
  v_ECI : Inport  Port=2
  Cross Product : matrix_library/Cross Product
  Cross Product1 : matrix_library/Cross Product
  Gain : Gain  Gain=-1
  Matrix Concatenate : Concatenate  NumInputs=3  Mode=Multidimensional array  ConcatenateDimension=2
  Normalize Vector : vrlib/Utilities/Normalize Vector  maxzero=0
  Normalize Vector1 : vrlib/Utilities/Normalize Vector  maxzero=0
  Transpose : Math  Operator=transpose
  DCM_ECI2orb : Outport
  wires:
  Matrix Concatenate/1 -> Transpose/1
  Normalize Vector1/1 -> Cross Product1/1, Matrix Concatenate/2  "y-axis"
  v_ECI/1 -> Cross Product/2
  Gain/1 -> Matrix Concatenate/3, Cross Product1/2  "z-axis"
  Cross Product/1 -> Normalize Vector1/1  "h = r x v"
  Normalize Vector/1 -> Gain/1
  Cross Product1/1 -> Matrix Concatenate/1  "x-axis"
  r_ECI/1 -> Normalize Vector/1, Cross Product/1
  Transpose/1 -> DCM_ECI2orb/1

== system TargetPosVel/Main/Environmental Torques/Magnetic Torque/Subsystem ==
  Xi : Inport
  Clock : Clock
  Demux : Demux  Outputs=3
  Direction Cosine Matrix ECEF to NED : aerolibtransform2/Direction Cosine Matrix ECEF to NED
  ECI Position to LLA : aerolibtransform2/ECI Position to LLA  red=IAU-2000/2006  year=yearValue  month=January  day=1  hour=hourValue  min=minuteValue  sec=secondValue  deltaT=Sec  errorflag=Warning  extraparamflag=off  eunits=Metric (MKS)  earthmodel=WGS84  flat=1/298.257223563  eqradius=6378137
      settings: AttributesFormatString=%<red>
  Gain : Gain  Gain=1e-9
  Matrix Multiply : Product  Multiplication=Matrix(*)
  Mux : Mux  Inputs=2
  Selector : Selector  InputPortWidth=3  IndexOptions=Index vector (dialog)  Indices=[3 1 2]  OutputSizes=1
  Transpose : Math  Operator=transpose
  World Magnetic Model : aerolibgravity2/World Magnetic Model  model=WMM2020 (2020-2025)  customFile='WMM2020.COF'  units=Metric (MKS)  time_in=off  month=January  day=1  year=yearValue  action=Error  h_out=off  dec_out=off  inc_out=off  ti_out=off
  MagField_ECEF : Outport
  wires:
  Matrix Multiply/1 -> MagField_ECEF/1
  Demux/3 -> Mux/2, World Magnetic Model/3
  ECI Position to LLA/1 -> Selector/1
  Mux/1 -> Direction Cosine Matrix ECEF to NED/1
  World Magnetic Model/1 -> Gain/1
  Transpose/1 -> Matrix Multiply/1  "DCM_NED2ECEF"
  Selector/1 -> Demux/1
  Gain/1 -> Matrix Multiply/2
  Demux/1 -> World Magnetic Model/1
  Direction Cosine Matrix ECEF to NED/1 -> Transpose/1
  Demux/2 -> Mux/1, World Magnetic Model/2
  Xi/1 -> ECI Position to LLA/1
  Clock/1 -> ?

== system TargetPosVel/Main/Subsystem/GPS/Subsystem ==
  LLA : Inport
  V_NED : Inport  Port=2
  Clock : Clock
  Demux : Demux  Outputs=3
  Direction Cosine Matrix ECEF to NED : aerolibtransform2/Direction Cosine Matrix ECEF to NED
  Direction Cosine Matrix ECI to ECEF : aerolibtransform2/Direction Cosine Matrix ECI to ECEF  red=IAU-2000/2006  year=yearValue  month=January  day=1  hour=hourValue  min=minuteValue  sec=secondValue  deltaT=Sec  errorflag=Error  extraparamflag=off
      settings: AttributesFormatString=%<red>
  LLA to ECI Position : aerolibtransform2/LLA to ECI Position  red=IAU-2000/2006  year=yearValue  month=January  day=1  hour=hourValue  min=minuteValue  sec=secondValue  deltaT=Sec  errorflag=Error  extraparamflag=off  eunits=Metric (MKS)  earthmodel=WGS84  flat=1/298.257223563  eqradius=6378137
      settings: AttributesFormatString=%<red>
  Mux : Mux  Inputs=2
  Product : Product  Multiplication=Matrix(*)
  Product2 : Product  Multiplication=Matrix(*)
  Terminator : Terminator
  Transpose : Math  Operator=transpose
  Transpose1 : Math  Operator=transpose
  X_GPS : Outport
  V_GPS : Outport  Port=2
  wires:
  LLA/1 -> Demux/1, LLA to ECI Position/1
  Clock/1 -> Direction Cosine Matrix ECI to ECEF/1, LLA to ECI Position/2
  LLA to ECI Position/1 -> X_GPS/1
  V_NED/1 -> Product/2
  Transpose1/1 -> Product2/1
  Direction Cosine Matrix ECI to ECEF/1 -> Transpose1/1
  Direction Cosine Matrix ECEF to NED/1 -> Transpose/1
  Product/1 -> Product2/2  "V_ECEF"
  Transpose/1 -> Product/1
  Product2/1 -> V_GPS/1
  Demux/3 -> Terminator/1
  Demux/1 -> Mux/1
  Demux/2 -> Mux/2
  Mux/1 -> Direction Cosine Matrix ECEF to NED/1

== system TargetPosVel/Main/Subsystem/GPS/Subsystem1 ==
  Xi : Inport
  Vi : Inport  Port=2
  t_JD : Inport  Port=3
  Clock : Clock
  Direction Cosine Matrix ECEF to NED : aerolibtransform2/Direction Cosine Matrix ECEF to NED
  ECI Position to LLA : aerolibtransform2/ECI Position to LLA  red=IAU-2000/2006  year=yearValue  month=January  day=1  hour=hourValue  min=minuteValue  sec=secondValue  deltaT=Sec  errorflag=Error  extraparamflag=off  eunits=Metric (MKS)  earthmodel=WGS84  flat=1/298.257223563  eqradius=6378137
      settings: AttributesFormatString=%<red>
  MATLAB Function : MATLAB Function  TreatAsAtomicUnit=on
  Product : Product  Multiplication=Matrix(*)
  Product1 : Product  Multiplication=Matrix(*)
  Selector : Selector  InputPortWidth=3  IndexOptions=Index vector (dialog)  Indices=[1 2]  OutputSizes=1
  v_NED : Outport
  wires:
  Xi/1 -> ECI Position to LLA/1
  Product/1 -> Product1/2
  ECI Position to LLA/1 -> Selector/1
  Direction Cosine Matrix ECEF to NED/1 -> Product1/1
  MATLAB Function/1(DCM_eci2ecef) -> Product/1
  Vi/1 -> Product/2
  Product1/1 -> v_NED/1
  Selector/1 -> Direction Cosine Matrix ECEF to NED/1
  t_JD/1 -> MATLAB Function/1(jd)
  Clock/1 -> ECI Position to LLA/2

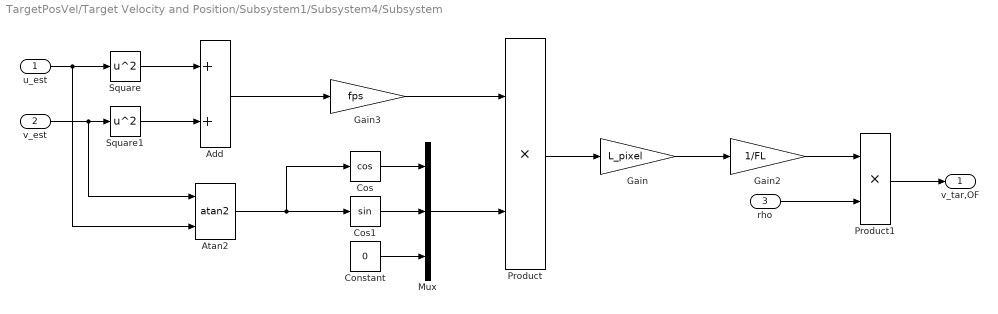
== system TargetPosVel/Target Velocity and Position/Subsystem1/Subsystem4/Subsystem ==
  u_est : Inport
  v_est : Inport  Port=2
  rho : Inport  Port=3
  Add : Sum
  Atan2 : Trigonometry  Operator=atan2
  Constant : Constant  Value=0
  Cos : Trigonometry  Operator=cos
  Cos1 : Trigonometry
  Gain : Gain  Gain=L_pixel
  Gain2 : Gain  Gain=1/FL
  Gain3 : Gain  Gain=fps
  Mux : Mux  Inputs=3
  Product : Product
  Product1 : Product
  Square : Math  Operator=square
  Square1 : Math  Operator=square
  v_tar,OF : Outport
  wires:
  u_est/1 -> Atan2/2, Square/1
  Add/1 -> Gain3/1
  Square/1 -> Add/1
  Square1/1 -> Add/2
  v_est/1 -> Square1/1, Atan2/1
  Atan2/1 -> Cos/1, Cos1/1
  Constant/1 -> Mux/3
  Cos/1 -> Mux/1
  Cos1/1 -> Mux/2
  Mux/1 -> Product/2
  Product/1 -> Gain/1
  Gain3/1 -> Product/1
  Gain/1 -> Gain2/1
  Gain2/1 -> Product1/1
  rho/1 -> Product1/2
  Product1/1 -> v_tar,OF/1

== system TargetPosVel/Target Velocity and Position/Subsystem1/Subsystem4/Subsystem1 ==
  vP : Inport
  rho : Inport  Port=2
  Constant : Constant  Value=1/fps
  Demux : Demux  Outputs=2
  Divide : Product  Inputs=*/
  Gain : Gain  Gain=1/L_pixel
  Gain1 : Gain  Gain=1/L_pixel
  Gain2 : Gain  Gain=FL
  Product : Product
  u : Outport
  v : Outport  Port=2
  wires:
  Demux/1 -> Gain/1
  Gain2/1 -> Divide/1
  Product/1 -> Demux/1
  Demux/2 -> Gain1/1
  Divide/1 -> Product/1
  Gain/1 -> u/1
  Constant/1 -> Product/2
  vP/1 -> Gain2/1
  rho/1 -> Divide/2
  Gain1/1 -> v/1

== system TargetPosVel/Target Velocity and Position/Subsystem8/Subsystem1/Subsystem ==
  Xi : Inport
  Clock : Clock
      settings: Decimation=1/timeStep
  Demux : Demux  Outputs=3
  ECI Position to LLA : aerolibtransform2/ECI Position to LLA  red=IAU-2000/2006  year=yearValue  month=January  day=1  hour=hourValue  min=minuteValue  sec=secondValue  deltaT=Sec  errorflag=Error  extraparamflag=off  eunits=Metric (MKS)  earthmodel=WGS84  flat=1/298.257223563  eqradius=6378137
      settings: AttributesFormatString=%<red>
  LLA to ECI Position : aerolibtransform2/LLA to ECI Position  red=IAU-2000/2006  year=yearValue  month=January  day=1  hour=hourValue  min=minuteValue  sec=secondValue  deltaT=Sec  errorflag=Error  extraparamflag=off  eunits=Metric (MKS)  earthmodel=WGS84  flat=1/298.257223563  eqradius=6378137
      settings: AttributesFormatString=%<red>
  MATLAB Function : MATLAB Function  TreatAsAtomicUnit=on
  Mux : Mux  Inputs=3
  Scope : Scope
  Scope1 : Scope
  Scope2 : Scope
  To File : ToFile  Filename=targetLLA.mat  MatrixName=targetLLA  SampleTime=timeStep
  rP_ECI : Outport
  wires:
  Xi/1 -> ECI Position to LLA/1
  Clock/1 -> LLA to ECI Position/2, ECI Position to LLA/2
  ECI Position to LLA/1 -> Demux/1
  Demux/1 -> Scope/1, Mux/1
  Demux/2 -> Scope1/1, Mux/2
  Demux/3 -> MATLAB Function/1(u)
  MATLAB Function/1(y) -> Scope2/1, Mux/3
  Mux/1 -> To File/1, LLA to ECI Position/1
  LLA to ECI Position/1 -> rP_ECI/1

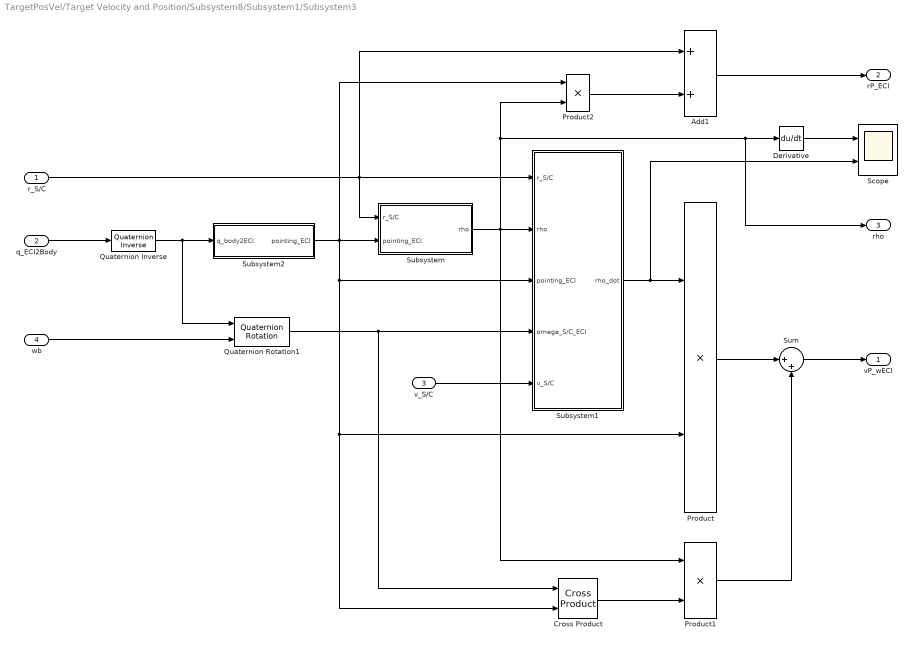
== system TargetPosVel/Target Velocity and Position/Subsystem8/Subsystem1/Subsystem3 ==
  r_S/C : Inport
  q_ECI2Body : Inport  Port=2
  v_S/C : Inport  Port=3
  wb : Inport  Port=4
  Add1 : Sum
  Cross Product : matrix_library/Cross Product
  Derivative : Derivative
  Product : Product
  Product1 : Product
  Product2 : Product
  Quaternion Inverse : aerolibutil/Quaternion Inverse
  Quaternion Rotation1 : aerolibutil/Quaternion Rotation
  Scope : Scope  NumInputPorts=2
  Subsystem : Subsystem
  Subsystem1 : Subsystem
  Subsystem2 : Subsystem
  Sum : Sum  Inputs=|++
  vP_wECI : Outport
  rP_ECI : Outport  Port=2
  rho : Outport  Port=3
  wires:
  Subsystem1/1(rho_dot) -> Scope/2, Product/1
  Sum/1 -> vP_wECI/1
  v_S/C/1 -> Subsystem1/5(v_S/C)
  Add1/1 -> rP_ECI/1
  Quaternion Inverse/1 -> Quaternion Rotation1/1, Subsystem2/1(q_body2ECI)
  q_ECI2Body/1 -> Quaternion Inverse/1
  r_S/C/1 -> Add1/1, Subsystem/1(r_S/C), Subsystem1/1(r_S/C)
  Subsystem/1(rho) -> Product2/2, rho/1, Derivative/1, Product1/1, Subsystem1/2(rho)
  Subsystem2/1(pointing_ECI) -> Product2/1, Subsystem/2(pointing_ECI), Product/2, Cross Product/2, Subsystem1/3(pointing_ECI)
  Product1/1 -> Sum/2
  Product2/1 -> Add1/2
  Cross Product/1 -> Product1/2
  Product/1 -> Sum/1
  Derivative/1 -> Scope/1
  wb/1 -> Quaternion Rotation1/2
  Quaternion Rotation1/1 -> Cross Product/1, Subsystem1/4(omega_S/C_ECI)

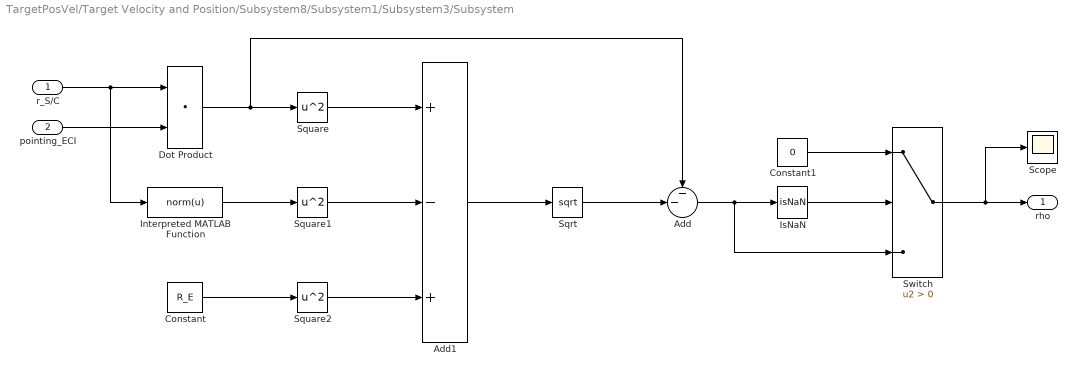
== system TargetPosVel/Target Velocity and Position/Subsystem8/Subsystem1/Subsystem3/Subsystem ==
  r_S/C : Inport
  pointing_ECI : Inport  Port=2
  Add : Sum  Inputs=--|
  Add1 : Sum  Inputs=+-+
  Constant : Constant  Value=R_E
  Constant1 : Constant  Value=0
  Dot Product : DotProduct  OutDataTypeStr=Inherit: Inherit via internal rule
  Interpreted MATLAB Function : MATLABFcn  MATLABFcn=norm(u)
  IsNaN : RelationalOperator  Operator=isNaN  OutDataTypeStr=boolean  RndMeth=Simplest  InputSameDT=off
  Scope : Scope
  Sqrt : Sqrt
  Square : Math  Operator=square
  Square1 : Math  Operator=square
  Square2 : Math  Operator=square
  Switch : Switch  Criteria=u2 > Threshold  SaturateOnIntegerOverflow=off  InputSameDT=off
  rho : Outport
  wires:
  Dot Product/1 -> Square/1, Add/1
  Square2/1 -> Add1/3
  Constant/1 -> Square2/1
  Square1/1 -> Add1/2
  Interpreted MATLAB Function/1 -> Square1/1
  Square/1 -> Add1/1
  Add1/1 -> Sqrt/1
  r_S/C/1 -> Dot Product/1, Interpreted MATLAB Function/1
  Constant1/1 -> Switch/1
  IsNaN/1 -> Switch/2
  Sqrt/1 -> Add/2
  Add/1 -> Switch/3, IsNaN/1
  pointing_ECI/1 -> Dot Product/2
  Switch/1 -> Scope/1, rho/1

== system TargetPosVel/Target Velocity and Position/Subsystem8/Subsystem1/Subsystem3/Subsystem1 ==
  r_S/C : Inport
  rho : Inport  Port=2
  pointing_ECI : Inport  Port=3
  omega_S/C_ECI : Inport  Port=4
  v_S/C : Inport  Port=5
  Add : Sum
  Add3 : Sum
  Cross Product : matrix_library/Cross Product
  Divide : Product  Inputs=*/
  Dot Product1 : DotProduct  OutDataTypeStr=Inherit: Inherit via internal rule
  Dot Product2 : DotProduct  OutDataTypeStr=Inherit: Inherit via internal rule
  Dot Product3 : DotProduct  OutDataTypeStr=Inherit: Inherit via internal rule
  Gain : Gain  Gain=-1
  Product : Product
  rho_dot : Outport
  wires:
  Gain/1 -> Product/1
  v_S/C/1 -> Dot Product2/2
  pointing_ECI/1 -> Dot Product2/1, Dot Product3/2, Cross Product/2
  Divide/1 -> rho_dot/1
  Dot Product2/1 -> Add/2
  Product/1 -> Divide/1
  r_S/C/1 -> Dot Product3/1, Dot Product1/1
  Dot Product3/1 -> Add3/2
  Cross Product/1 -> Dot Product1/2
  rho/1 -> Add3/1, Gain/1
  Dot Product1/1 -> Add/1
  Add/1 -> Product/2
  Add3/1 -> Divide/2
  omega_S/C_ECI/1 -> Cross Product/1

== system TargetPosVel/Target Velocity and Position/Subsystem8/Subsystem1/Subsystem3/Subsystem2 ==
  q_body2ECI : Inport
  Constant : Constant  Value=pointing_body
  Quaternion Rotation : aerolibutil/Quaternion Rotation
  pointing_ECI : Outport
  wires:
  Constant/1 -> Quaternion Rotation/2
  q_body2ECI/1 -> Quaternion Rotation/1
  Quaternion Rotation/1 -> pointing_ECI/1

== matlab function TargetPosVel/Target Velocity and Position/Subsystem1/Subsystem4/MATLAB Function ==
  data: img input size=[1200,1920,3]; u input size=1; original_img output size=[1200,1920,3]; v input size=1; shifted_img output size=[1200,1920,3]
function [original_img, shifted_img] = img_shift(img, u, v)

shifted_img  = imtranslate(img, [u,v]);
original_img = img;

end

== matlab function TargetPosVel/Target Velocity and Position/Subsystem8/Subsystem1/Subsystem/MATLAB Function ==
  data: u input; y output
function y = fcn(u)

y = u;

% We need to force the altitude to be a non-negative number because in the
% model we assumed a spherical Earth while the Simulink conversion block 
% assumes the WGS84 Earth model.
for i = 1:length(y)
    if y(i) < 0
        y(i) = 0;
    end
end

end
